simulink subsystem "SimpleEngine"  (R2023a)
settings: Solver=VariableStepAuto  StartTime=0.0  StopTime=10.0  RelTol=1e-3
libraries: autolibhevctrlrcommon x1, autolibpowerinfoutils x1, autolibsharedmappedengines x1, autolibutils x1
settings Model: ModifiedByFormat=The MathWorks, Inc.  Creator=The MathWorks, Inc.  LastModifiedBy=The MathWorks, Inc.
settings SolverCC: MaxZcPerStep=1
settings OptimizationCC: ReuseModelBlockBuffer=off
settings DebuggingCC: UnconnectedInputMsg=warning  UnconnectedOutputMsg=warning  UnconnectedLineMsg=warning
settings ModelReferenceCC: EnableRefExpFcnMdlSchedulingChecks=on
settings RTWCC: DLArmComputeVersion=19.05

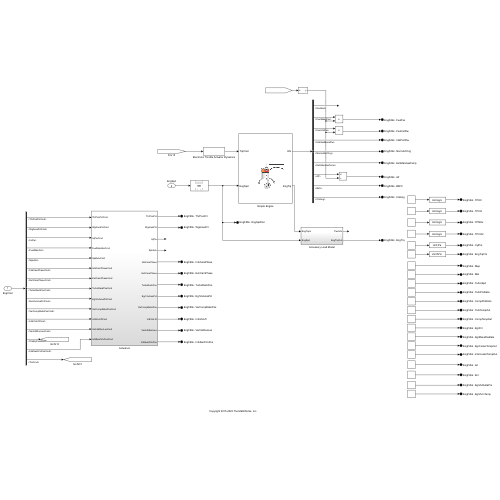
[thumbnail: Simulink's stored preview of the top-level diagram]
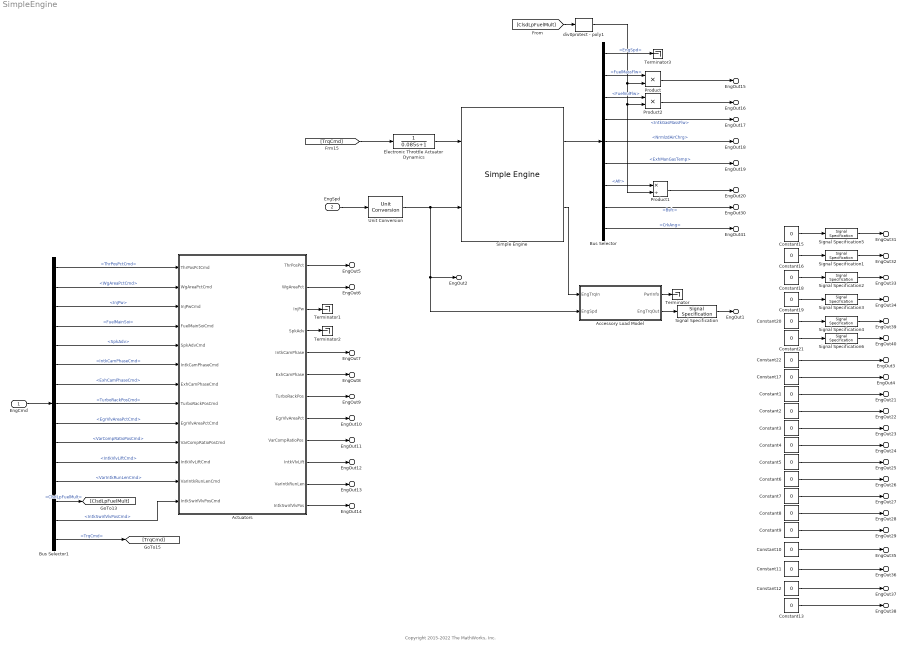
== system SimpleEngine ==
  note: Copyright 2015-2022 The MathWorks, Inc.
  EngCmd : Inport
  EngSpd : Inport  Port=2  Unit=rad/sec
  Accessory Load Model : Subsystem
  Actuators : Subsystem
  Bus Selector : BusSelector  OutputSignals=EngSpd,FuelMassFlw,FuelVolFlw,IntkGasMassFlw,NrmlzdAirChrg,ExhManGasTemp,Afr,Bsfc,CrkAng
  Bus Selector1 : BusSelector  OutputSignals=ThrPosPctCmd,WgAreaPctCmd,InjPw,FuelMainSoi,SpkAdv,IntkCamPhaseCmd,ExhCamPhaseCmd,TurboRackPosCmd,EgrVlvAreaPctCmd,VarCompRatioPosCmd,IntkVlvLiftCmd,VarIntkRunLenCmd,ClsdLpFuelMult,IntkSwirlVlvPosCmd,TrqCmd
  Constant{1..13,15..22} (21 alike) : Constant  Value=0  SampleTime=-1
  Electronic Throttle Actuator Dynamics : TransferFcn  Denominator=[0.085 1]
  Product : Product
  Product1 : Product  Inputs=*/
  Product2 : Product
  Signal Specification : SignalSpecification  Dimensions=1
  Signal Specification{1..3,5} (4 alike) : SignalSpecification  Unit=kg/s
  Signal Specification4 : SignalSpecification  Unit=Pa
  Signal Specification6 : SignalSpecification  Unit=N*m
  Simple Engine : autolibsharedmappedengines/Simple Engine  f_tqmax=PlntEngTqMax  f_tqmax_n_bpt=PlntEngTqMaxBpt  Lhv=PlntEngLhv  Sg=PlntEngSg  BsfcAvg=PlntEngBsfcAvg  aMode=6
  Terminator{,1..3} (4 alike) : Terminator
  Unit Conversion : UnitConversion
  div0protect - poly1 : autolibutils/div0protect - poly  thresh=0.01  ZeroCross1=off  aMode=6
  EngOut1 : Outport  PortName=EngFdbk  Element=EngTrq
  EngOut2 : Outport  PortName=EngFdbk  Element=EngSpdOut
  EngOut3 : Outport  PortName=EngFdbk  Element=Map
  EngOut4 : Outport  PortName=EngFdbk  Element=Mat
  EngOut5 : Outport  PortName=EngFdbk  Element=ThrPosPct
  EngOut6 : Outport  PortName=EngFdbk  Element=WgAreaPct
  EngOut7 : Outport  PortName=EngFdbk  Element=IntkCamPhase
  EngOut8 : Outport  PortName=EngFdbk  Element=ExhCamPhase
  EngOut9 : Outport  PortName=EngFdbk  Element=TurboRackPos
  EngOut10 : Outport  PortName=EngFdbk  Element=EgrVlvAreaPct
  EngOut11 : Outport  PortName=EngFdbk  Element=VarCompRatioPos
  EngOut12 : Outport  PortName=EngFdbk  Element=IntkVlvLift
  EngOut13 : Outport  PortName=EngFdbk  Element=VarIntkRunLen
  EngOut14 : Outport  PortName=EngFdbk  Element=IntkSwirlVlvPos
  EngOut15 : Outport  PortName=EngFdbk  Element=FuelFlw
  EngOut16 : Outport  PortName=EngFdbk  Element=FuelVolFlw
  EngOut17 : Outport  PortName=EngFdbk  Element=IntkPortFlw
  EngOut18 : Outport  PortName=EngFdbk  Element=NormAirChrg
  EngOut19 : Outport  PortName=EngFdbk  Element=ExhManGasTemp
  EngOut20 : Outport  PortName=EngFdbk  Element=Afr
  EngOut21 : Outport  PortName=EngFdbk  Element=TurboSpd
  EngOut22 : Outport  PortName=EngFdbk  Element=TurbPrsRatio
  EngOut23 : Outport  PortName=EngFdbk  Element=CompPrsRatio
  EngOut24 : Outport  PortName=EngFdbk  Element=TurbTempOut
  EngOut25 : Outport  PortName=EngFdbk  Element=CompTempOut
  EngOut26 : Outport  PortName=EngFdbk  Element=EgrPct
  EngOut27 : Outport  PortName=EngFdbk  Element=EgrMassFlwRate
  EngOut28 : Outport  PortName=EngFdbk  Element=EgrCoolerTempOut
  EngOut29 : Outport  PortName=EngFdbk  Element=IntercoolerTempOut
  EngOut30 : Outport  PortName=EngFdbk  Element=BSFC
  EngOut31 : Outport  PortName=EngFdbk  Element=TPHC
  EngOut32 : Outport  PortName=EngFdbk  Element=TPCO
  EngOut33 : Outport  PortName=EngFdbk  Element=TPNOx
  EngOut34 : Outport  PortName=EngFdbk  Element=TPCO2
  EngOut35 : Outport  PortName=EngFdbk  Element=Iat
  EngOut36 : Outport  PortName=EngFdbk  Element=Ect
  EngOut37 : Outport  PortName=EngFdbk  Element=EgrVlvDeltaPrs
  EngOut38 : Outport  PortName=EngFdbk  Element=EgrVlvInTemp
  EngOut39 : Outport  PortName=EngFdbk  Element=CylPrs
  EngOut40 : Outport  PortName=EngFdbk  Element=EngTrqCrk
  EngOut41 : Outport  PortName=EngFdbk  Element=CrkAng
  wires:
  EngCmd/1 -> Bus Selector1/1
  Bus Selector1/3 -> Actuators/3(InjPwCmd)  "<InjPw>"
  Bus Selector1/1 -> Actuators/1(ThrPosPctCmd)  "<ThrPosPctCmd>"
  Bus Selector1/2 -> Actuators/2(WgAreaPctCmd)  "<WgAreaPctCmd>"
  Bus Selector1/11 -> Actuators/11(IntkVlvLiftCmd)  "<IntkVlvLiftCmd>"
  Bus Selector1/4 -> Actuators/4(FuelMainSoiCmd)  "<FuelMainSoi>"
  Bus Selector1/7 -> Actuators/7(ExhCamPhaseCmd)  "<ExhCamPhaseCmd>"
  Bus Selector1/9 -> Actuators/9(EgrVlvAreaPctCmd)  "<EgrVlvAreaPctCmd>"
  Bus Selector1/12 -> Actuators/12(VarIntkRunLenCmd)  "<VarIntkRunLenCmd>"
  Bus Selector1/5 -> Actuators/5(SpkAdvCmd)  "<SpkAdv>"
  Bus Selector1/6 -> Actuators/6(IntkCamPhaseCmd)  "<IntkCamPhaseCmd>"
  Bus Selector1/8 -> Actuators/8(TurboRackPosCmd)  "<TurboRackPosCmd>"
  Bus Selector1/10 -> Actuators/10(VarCompRatioPosCmd)  "<VarCompRatioPosCmd>"
  Bus Selector1/15 -> [TrqCmd]  "<TrqCmd>"
  Bus Selector1/14 -> Actuators/13(IntkSwirlVlvPosCmd)  "<IntkSwirlVlvPosCmd>"
  Bus Selector1/13 -> [ClsdLpFuelMult]  "<ClsdLpFuelMult>"
  Constant16/1 -> Signal Specification1/1
  Constant9/1 -> EngOut29/1
  Simple Engine/2 -> Accessory Load Model/1(EngTrqIn)
  Bus Selector/9 -> EngOut41/1  "<CrkAng>"
  Bus Selector/1 -> Terminator3/1  "<EngSpd>"
  Actuators/1(ThrPosPct) -> EngOut5/1
  Actuators/11(VarIntkRunLen) -> EngOut13/1
  Constant5/1 -> EngOut25/1
  Product/1 -> EngOut15/1
  Constant21/1 -> Signal Specification6/1
  Constant19/1 -> Signal Specification3/1
  Bus Selector/6 -> EngOut19/1  "<ExhManGasTemp>"
  Constant17/1 -> EngOut4/1
  [ClsdLpFuelMult] -> div0protect - poly1/1
  Constant6/1 -> EngOut26/1
  EngSpd/1 -> Unit Conversion/1
  Constant2/1 -> EngOut22/1
  Actuators/6(ExhCamPhase) -> EngOut8/1
  Accessory Load Model/2(EngTrqOut) -> Signal Specification/1
  Bus Selector/5 -> EngOut18/1  "<NrmlzdAirChrg>"
  div0protect - poly1/1 -> Product/2, Product1/2, Product2/2
  Signal Specification4/1 -> EngOut39/1
  Constant20/1 -> Signal Specification4/1
  Actuators/5(IntkCamPhase) -> EngOut7/1
  Constant12/1 -> EngOut37/1
  Accessory Load Model/1(PwrInfo) -> Terminator/1
  Constant22/1 -> EngOut3/1
  Actuators/8(EgrVlvAreaPct) -> EngOut10/1
  Bus Selector/3 -> Product2/1  "<FuelVolFlw>"
  Actuators/9(VarCompRatioPos) -> EngOut11/1
  Constant7/1 -> EngOut27/1
  [TrqCmd] -> Electronic Throttle Actuator Dynamics/1
  Constant18/1 -> Signal Specification2/1
  Actuators/10(IntkVlvLift) -> EngOut12/1
  Actuators/3(InjPw) -> Terminator1/1
  Product1/1 -> EngOut20/1
  Bus Selector/4 -> EngOut17/1  "<IntkGasMassFlw>"
  Actuators/12(IntkSwirlVlvPos) -> EngOut14/1
  Bus Selector/7 -> Product1/1  "<Afr>"
  Constant4/1 -> EngOut24/1
  Actuators/2(WgAreaPct) -> EngOut6/1
  Bus Selector/2 -> Product/1  "<FuelMassFlw>"
  Constant11/1 -> EngOut36/1
  Constant3/1 -> EngOut23/1
  Electronic Throttle Actuator Dynamics/1 -> Simple Engine/1
  Constant8/1 -> EngOut28/1
  Signal Specification1/1 -> EngOut32/1
  Actuators/7(TurboRackPos) -> EngOut9/1
  Constant13/1 -> EngOut38/1
  Signal Specification5/1 -> EngOut31/1
  Actuators/4(SpkAdv) -> Terminator2/1
  Signal Specification2/1 -> EngOut33/1
  Constant1/1 -> EngOut21/1
  Product2/1 -> EngOut16/1
  Constant10/1 -> EngOut35/1
  Signal Specification3/1 -> EngOut34/1
  Simple Engine/1 -> Bus Selector/1
  Bus Selector/8 -> EngOut30/1  "<Bsfc>"
  Constant15/1 -> Signal Specification5/1
  Signal Specification6/1 -> EngOut40/1
  Unit Conversion/1 -> Accessory Load Model/2(EngSpd), EngOut2/1, Simple Engine/2
  Signal Specification/1 -> EngOut1/1

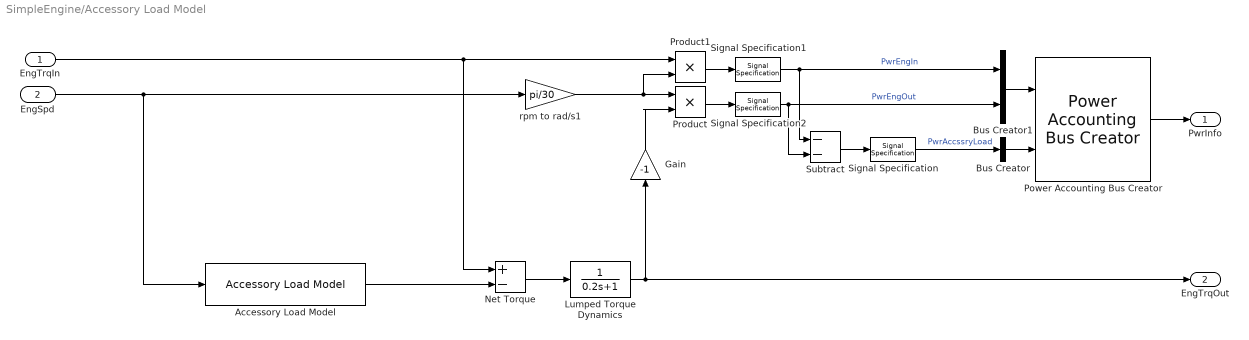
== system SimpleEngine/Accessory Load Model ==
  EngTrqIn : Inport
  EngSpd : Inport  Port=2
  Accessory Load Model : autolibhevctrlrcommon/Accessory Load Model  AccPwrTbl=PlntEngAccPwrTbl  AccSpdBpts=PlntEngAccSpdBpt
  Bus Creator : BusCreator  Inputs=1
  Bus Creator1 : BusCreator  Inputs=2
  Gain : Gain  Gain=-1
  Lumped Torque Dynamics : TransferFcn  Denominator=[0.2 1]
  Net Torque : Sum  Inputs=+-
  Power Accounting Bus Creator : autolibpowerinfoutils/Power Accounting Bus Creator  AssctBlkSelPopup=Parent  RefBlkName='libraryname/blkname'  PwrTrnsfrdCheckBox=on  PwrNotTrnsfrdCheckBox=on  PwrStoredCheckBox=off  aMode=6
      settings: SourceProductName=Powertrain Blockset
  Product : Product
  Product1 : Product
  Signal Specification : SignalSpecification  Unit=W
  Signal Specification1 : SignalSpecification  Unit=W
  Signal Specification2 : SignalSpecification  Unit=W
  Subtract : Sum  Inputs=--
  rpm to rad/s1 : Gain  Gain=pi/30
  PwrInfo : Outport  VectorParamsAs1DForOutWhenUnconnected=off
  EngTrqOut : Outport  Port=2  Unit=N*m  VectorParamsAs1DForOutWhenUnconnected=off
  wires:
  Gain/1 -> Product/2
  Signal Specification2/1 -> Bus Creator1/2, Subtract/2  "PwrEngOut"
  Signal Specification1/1 -> Bus Creator1/1, Subtract/1  "PwrEngIn"
  rpm to rad/s1/1 -> Product/1, Product1/2
  Product1/1 -> Signal Specification1/1
  Product/1 -> Signal Specification2/1
  Power Accounting Bus Creator/1 -> PwrInfo/1
  Signal Specification/1 -> Bus Creator/1  "PwrAccssryLoad"
  Subtract/1 -> Signal Specification/1
  EngTrqIn/1 -> Net Torque/1, Product1/1
  Bus Creator1/1 -> Power Accounting Bus Creator/1
  Bus Creator/1 -> Power Accounting Bus Creator/2
  Net Torque/1 -> Lumped Torque Dynamics/1
  Lumped Torque Dynamics/1 -> Gain/1, EngTrqOut/1
  EngSpd/1 -> rpm to rad/s1/1, Accessory Load Model/1
  Accessory Load Model/1 -> Net Torque/2

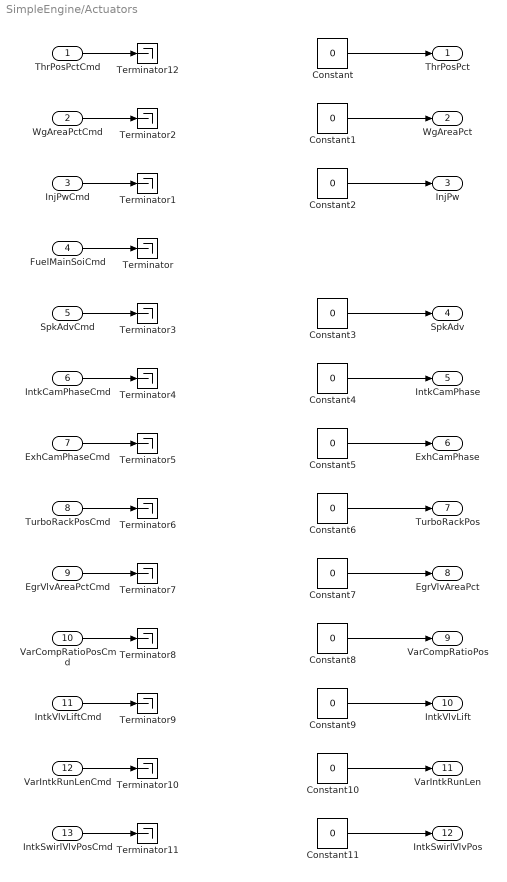
== system SimpleEngine/Actuators ==
  ThrPosPctCmd : Inport  Unit=%
  WgAreaPctCmd : Inport  Port=2  Unit=%
  InjPwCmd : Inport  Port=3  Unit=ms
  FuelMainSoiCmd : Inport  Port=4  Unit=deg
  SpkAdvCmd : Inport  Port=5  Unit=deg
  IntkCamPhaseCmd : Inport  Port=6  Unit=deg
  ExhCamPhaseCmd : Inport  Port=7  Unit=deg
  TurboRackPosCmd : Inport  Port=8  Unit=1
  EgrVlvAreaPctCmd : Inport  Port=9  Unit=%
  VarCompRatioPosCmd : Inport  Port=10
  IntkVlvLiftCmd : Inport  Port=11
  VarIntkRunLenCmd : Inport  Port=12
  IntkSwirlVlvPosCmd : Inport  Port=13
  Constant{,1..11} (12 alike) : Constant  Value=0  SampleTime=-1
  Terminator{,1..12} (13 alike) : Terminator
  ThrPosPct : Outport  Unit=%  VectorParamsAs1DForOutWhenUnconnected=off
  WgAreaPct : Outport  Port=2  Unit=%  VectorParamsAs1DForOutWhenUnconnected=off
  InjPw : Outport  Port=3  VectorParamsAs1DForOutWhenUnconnected=off
  SpkAdv : Outport  Port=4  VectorParamsAs1DForOutWhenUnconnected=off
  IntkCamPhase : Outport  Port=5  Unit=deg  VectorParamsAs1DForOutWhenUnconnected=off
  ExhCamPhase : Outport  Port=6  Unit=deg  VectorParamsAs1DForOutWhenUnconnected=off
  TurboRackPos : Outport  Port=7  Unit=1  VectorParamsAs1DForOutWhenUnconnected=off
  EgrVlvAreaPct : Outport  Port=8  Unit=%  VectorParamsAs1DForOutWhenUnconnected=off
  VarCompRatioPos : Outport  Port=9  VectorParamsAs1DForOutWhenUnconnected=off
  IntkVlvLift : Outport  Port=10  VectorParamsAs1DForOutWhenUnconnected=off
  VarIntkRunLen : Outport  Port=11  VectorParamsAs1DForOutWhenUnconnected=off
  IntkSwirlVlvPos : Outport  Port=12  VectorParamsAs1DForOutWhenUnconnected=off
  wires:
  Constant9/1 -> IntkVlvLift/1
  Constant10/1 -> VarIntkRunLen/1
  Constant11/1 -> IntkSwirlVlvPos/1
  Constant8/1 -> VarCompRatioPos/1
  Constant7/1 -> EgrVlvAreaPct/1
  Constant6/1 -> TurboRackPos/1
  Constant3/1 -> SpkAdv/1
  Constant4/1 -> IntkCamPhase/1
  Constant5/1 -> ExhCamPhase/1
  Constant2/1 -> InjPw/1
  Constant1/1 -> WgAreaPct/1
  Constant/1 -> ThrPosPct/1
  SpkAdvCmd/1 -> Terminator3/1
  EgrVlvAreaPctCmd/1 -> Terminator7/1
  TurboRackPosCmd/1 -> Terminator6/1
  InjPwCmd/1 -> Terminator1/1
  VarIntkRunLenCmd/1 -> Terminator10/1
  VarCompRatioPosCmd/1 -> Terminator8/1
  IntkCamPhaseCmd/1 -> Terminator4/1
  ExhCamPhaseCmd/1 -> Terminator5/1
  ThrPosPctCmd/1 -> Terminator12/1
  WgAreaPctCmd/1 -> Terminator2/1
  IntkSwirlVlvPosCmd/1 -> Terminator11/1
  IntkVlvLiftCmd/1 -> Terminator9/1
  FuelMainSoiCmd/1 -> Terminator/1
